simulink model "Sim3e_merged"  (R2016a)
settings: Solver=VariableStepAuto  StartTime=0.0  StopTime=total_time  RelTol=1e-3
values from neighbouring files (symbols this model uses):
  A = [-0.322 0.052 0.028 -1.12   0.002 ... (first row only)    [Copy_of_modelParms.m]    (also in modelParms.m)
  antiWindupBound = 0.05    [Copy_of_modelParms.m]    (also in modelParms.m)
  B = [0 0 0 0 10]'    [Copy_of_modelParms.m]    (also in modelParms.m)
  C = [0 0 0 1 0 ... (first row only)    [Copy_of_modelParms.m]    (also in modelParms.m)
  dist = deg2rad(2)    [Copy_of_modelParms.m]    (also in modelParms.m)
  g = 9.8    [Copy_of_modelParms.m]    (also in modelParms.m)
  Gamma_k = Gamma    [Copy_of_modelParms.m]
  H_k = C_kalman    [Copy_of_modelParms.m]
  h_meas = .01    (= 0.01)    [modelParms.m]
  k_d_phi = (2*zeta_phi*omega_n_phi - alpha_phi1)/alpha_phi2    [Copy_of_modelParms.m]    (also in modelParms.m)
  k_i_chi = omega_n_chi^2*V_g/g    [Copy_of_modelParms.m]    (also in modelParms.m)
  k_p_chi = 2*zeta_chi*omega_n_chi*V_g/g    [Copy_of_modelParms.m]    (also in modelParms.m)
  k_p_phi = delta_a_max/e_phi_max * sign(alpha_phi2)    [Copy_of_modelParms.m]    (also in modelParms.m)
  P_bar_0 = Q    [Copy_of_modelParms.m]
  p_var = 0.5    [modelParms.m]
  Phi_k = Phi    [Copy_of_modelParms.m]
  phi_var = 2    [modelParms.m]
  Q_k = Q    [Copy_of_modelParms.m]
  R_k = R    [Copy_of_modelParms.m]
  r_var = 0.2    [modelParms.m]
  V_g = 637 * 1000 / 3600    (= 176.944444444)    [Copy_of_modelParms.m]    (also in modelParms.m)
  x_bar_0 = [0, 0, 0, 0]'    [Copy_of_modelParms.m]
undefined symbols (not defined in the file or in its folder): Delta_k
libraries: simulink x1
settings Model: Creator=Alex  LastModifiedBy=Alex

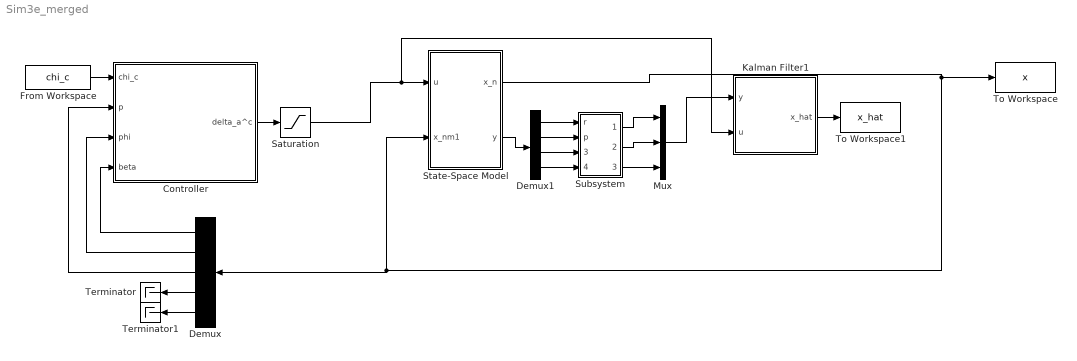
== system Sim3e_merged ==
  Controller : Subsystem
  Demux : Demux  Outputs=5
  Demux1 : Demux
  From Workspace : FromWorkspace  VariableName=chi_c  SampleTime=0
  Kalman Filter1 : Subsystem
  Mux : Mux  Inputs=3
  Saturation : Saturate  UpperLimit=deg2rad(25)  LowerLimit=deg2rad(-25)
  State-Space Model : Subsystem
  Subsystem : Subsystem
  Terminator : Terminator
  Terminator1 : Terminator
  To Workspace : ToWorkspace  VariableName=x  SaveFormat=Timeseries  SampleTime=-1
  To Workspace1 : ToWorkspace  VariableName=x_hat  SaveFormat=Timeseries  SampleTime=-1
  wires:
  Controller/1(delta_a^c) -> Saturation/1
  Demux/1 -> Controller/4(beta)
  Demux/2 -> Controller/3(phi)
  Demux/4 -> Terminator/1
  Demux/5 -> Terminator1/1
  Demux/3 -> Controller/2(p)
  From Workspace/1 -> Controller/1(chi_c)
  State-Space Model/1(x_n) -> State-Space Model/2(x_nm1), Demux/1, To Workspace/1
  State-Space Model/2(y) -> Demux1/1
  Mux/1 -> Kalman Filter1/1(y)
  Kalman Filter1/1(x_hat) -> To Workspace1/1
  Saturation/1 -> Kalman Filter1/2(u), State-Space Model/1(u)
  Demux1/1 -> Subsystem/1(r)
  Demux1/2 -> Subsystem/2(p)
  Demux1/3 -> Subsystem/3(beta)
  Demux1/4 -> Subsystem/4("phi ")
  Subsystem/1(r_meas) -> Mux/1
  Subsystem/2(p_meas) -> Mux/2
  Subsystem/3(phi_meas) -> Mux/3

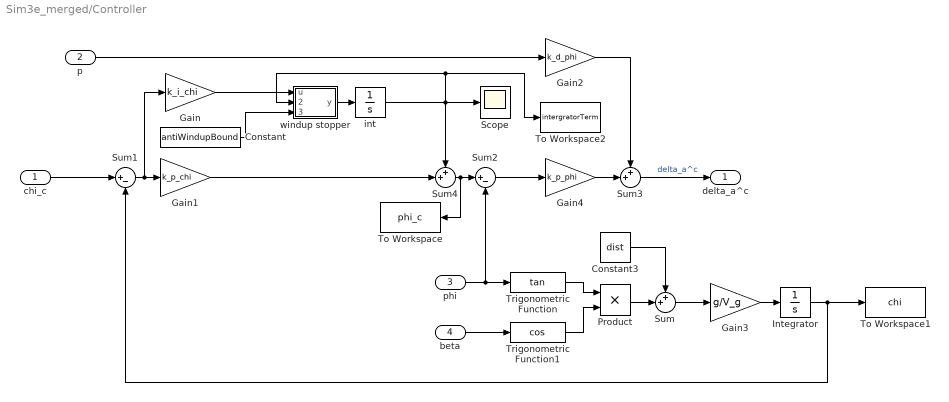
== system Sim3e_merged/Controller ==
  chi_c : Inport
  p : Inport  Port=2
  phi : Inport  Port=3
  beta : Inport  Port=4
  Constant : Constant  Value=antiWindupBound
  Constant3 : Constant  Value=dist
  Gain : Gain  Gain=k_i_chi
  Gain1 : Gain  Gain=k_p_chi
  Gain2 : Gain  Gain=k_d_phi
  Gain3 : Gain  Gain=g/V_g
  Gain4 : Gain  Gain=k_p_phi
  Integrator : Integrator
  Product : Product
  Scope : Scope
  Sum : Sum  Inputs=++|
  Sum1 : Sum  Inputs=|+-
  Sum2 : Sum  Inputs=|+-
  Sum3 : Sum  Inputs=++|
  Sum4 : Sum  Inputs=++|
  To Workspace : ToWorkspace  VariableName=phi_c  SaveFormat=Timeseries  SampleTime=-1
  To Workspace1 : ToWorkspace  VariableName=chi  SaveFormat=Timeseries  SampleTime=-1
  To Workspace2 : ToWorkspace  VariableName=intergratorTerm  SaveFormat=Timeseries  SampleTime=-1
  Trigonometric Function : Trigonometry  Operator=tan
  Trigonometric Function1 : Trigonometry  Operator=cos
  int : Integrator
  windup stopper : MATLAB Function  TreatAsAtomicUnit=on
  delta_a^c : Outport
  wires:
  Sum3/1 -> delta_a^c/1  "delta_a^c"
  Gain3/1 -> Integrator/1
  Trigonometric Function1/1 -> Product/2
  Trigonometric Function/1 -> Product/1
  beta/1 -> Trigonometric Function1/1
  Gain4/1 -> Sum3/2
  Sum4/1 -> To Workspace/1, Sum2/1
  p/1 -> Gain2/1
  chi_c/1 -> Sum1/1
  Gain1/1 -> Sum4/2
  Sum1/1 -> Gain1/1, Gain/1
  Sum2/1 -> Gain4/1
  Gain2/1 -> Sum3/1
  int/1 -> Scope/1, windup stopper/2(compare), To Workspace2/1, Sum4/1
  phi/1 -> Sum2/2, Trigonometric Function/1
  Integrator/1 -> Sum1/2, To Workspace1/1
  Gain/1 -> windup stopper/1(u)
  windup stopper/1(y) -> int/1
  Constant/1 -> windup stopper/3(antiWindupBound)
  Product/1 -> Sum/2
  Constant3/1 -> Sum/1
  Sum/1 -> Gain3/1

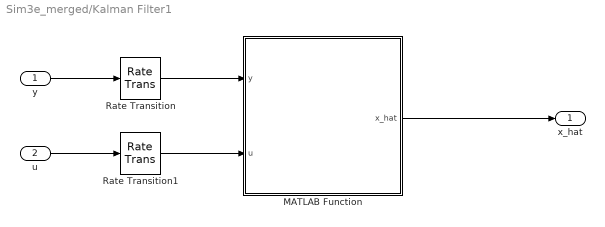
== system Sim3e_merged/Kalman Filter1 ==
  y : Inport
  u : Inport  Port=2
  MATLAB Function : MATLAB Function  TreatAsAtomicUnit=on
  Rate Transition : RateTransition  OutPortSampleTime=h
  Rate Transition1 : RateTransition  OutPortSampleTime=h
  x_hat : Outport
  wires:
  Rate Transition1/1 -> MATLAB Function/2(u)
  Rate Transition/1 -> MATLAB Function/1(y)
  u/1 -> Rate Transition1/1
  y/1 -> Rate Transition/1
  MATLAB Function/1(x_hat) -> x_hat/1

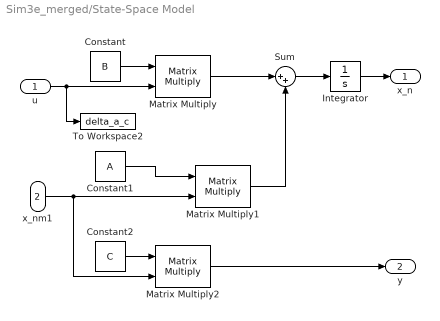
== system Sim3e_merged/State-Space Model ==
  u : Inport
  x_nm1 : Inport  Port=2
  Constant : Constant  Value=B
  Constant1 : Constant  Value=A
  Constant2 : Constant  Value=C
  Integrator : Integrator
  Matrix Multiply : Product  Multiplication=Matrix(*)
  Matrix Multiply1 : Product  Multiplication=Matrix(*)
  Matrix Multiply2 : Product  Multiplication=Matrix(*)
  Sum : Sum  Inputs=|++
  To Workspace2 : ToWorkspace  VariableName=delta_a_c  SaveFormat=Timeseries  SampleTime=-1
  x_n : Outport
  y : Outport  Port=2
  wires:
  Constant1/1 -> Matrix Multiply1/1
  Sum/1 -> Integrator/1
  Constant/1 -> Matrix Multiply/1
  u/1 -> To Workspace2/1, Matrix Multiply/2
  Integrator/1 -> x_n/1
  Matrix Multiply1/1 -> Sum/2
  Matrix Multiply/1 -> Sum/1
  x_nm1/1 -> Matrix Multiply1/2, Matrix Multiply2/2
  Constant2/1 -> Matrix Multiply2/1
  Matrix Multiply2/1 -> y/1

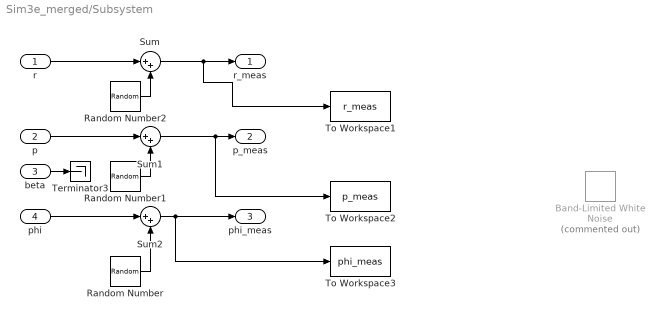
== system Sim3e_merged/Subsystem ==
  r : Inport
  p : Inport  Port=2
  beta : Inport  Port=3
  "phi " : Inport  Port=4
  Band-Limited White Noise : simulink/Sources/Band-Limited White Noise  Commented=on  Cov=deg2rad(deg2rad(r_var))*h_meas  Ts=h_meas  seed=[23341]
  Random Number : RandomNumber  Variance=deg2rad(deg2rad(phi_var))  SampleTime=h_meas
  Random Number1 : RandomNumber  Variance=deg2rad(deg2rad(p_var))  SampleTime=h_meas
  Random Number2 : RandomNumber  Variance=deg2rad(deg2rad(r_var))  SampleTime=h_meas
  Sum : Sum  Inputs=|++
  Sum1 : Sum  Inputs=|++
  Sum2 : Sum  Inputs=|++
  Terminator3 : Terminator
  To Workspace1 : ToWorkspace  VariableName=r_meas  SaveFormat=Timeseries  SampleTime=-1
  To Workspace2 : ToWorkspace  VariableName=p_meas  SaveFormat=Timeseries  SampleTime=-1
  To Workspace3 : ToWorkspace  VariableName=phi_meas  SaveFormat=Timeseries  SampleTime=-1
  r_meas : Outport
  p_meas : Outport  Port=2
  phi_meas : Outport  Port=3
  wires:
  Random Number1/1 -> Sum1/2
  "phi "/1 -> Sum2/1
  p/1 -> Sum1/1
  Random Number/1 -> Sum2/2
  r/1 -> Sum/1
  Sum/1 -> To Workspace1/1, r_meas/1
  Sum1/1 -> p_meas/1, To Workspace2/1
  beta/1 -> Terminator3/1
  Sum2/1 -> To Workspace3/1, phi_meas/1
  Random Number2/1 -> Sum/2

== matlab function Sim3e_merged/Controller/windup stopper ==
  data: u input; y output; compare input; antiWindupBound input
function y = fcn(u,compare, antiWindupBound)
%#codegen
if((abs(compare) >= antiWindupBound) && sign(u) == sign(compare))
    y = 0;
else
    y=u;
end

== matlab function Sim3e_merged/Kalman Filter1/MATLAB Function ==
  data: y input; u input; x_hat output; x_bar_0 parameter; P_bar_0 parameter; Phi_k parameter; Delta_k parameter; Gamma_k parameter; H_k parameter; Q_k parameter; R_k parameter
function x_hat = fcn(y, u, x_bar_0, P_bar_0, Phi_k, Delta_k, Gamma_k, H_k, Q_k, R_k)

persistent P_hat_k;                                                 % Error covariance
persistent P_bar_k;                                                 % Error covariance prediction
persistent K_k;                                                     % Kalman gain matrix
persistent x_bar_k;                                                 % State prediction
persistent k;                                                       % Time step
persistent I;                                                       % Identity matrix with correct dimensions

if(isempty(k))
    % Initialize
    k = 0;                                                          % Time step zero
    P_bar_k = P_bar_0;                                              % Initial error covariance
    x_bar_k = x_bar_0;                                              % Initial state estimate
    I = eye(length(P_bar_0));
else
    % Iterate
    k = k + 1;                                                      % Time step
end

% Correction
K_k = P_bar_k*(H_k')/(H_k*P_bar_k*(H_k')+R_k);                           % Kalman gain matrix
x_hat_k = x_bar_k + K_k*(y + H_k*x_bar_k);                          % State error update
P_hat_k = (I - K_k*H_k)*P_bar_k*((I-K_k*H_k)') + K_k*R_k*(K_k');  % Error covariance update

% Prediction
x_bar_k_pluss_one = Phi_k*x_hat_k + Delta_k*u;                      % State prediction
P_bar_k_pluss_one = Phi_k*P_hat_k*(Phi_k') + Gamma_k*Q_k*(Gamma_k');% Error covariance prediction

% Propagation
x_bar_k = x_bar_k_pluss_one;                                        % State estimate propagation
P_bar_k = P_bar_k_pluss_one;                                        % Error covariance propagation

% State estimate output
x_hat = x_hat_k;
